simulink library "hdlcoderNFPCast"  (R2019a)
settings: Solver=VariableStepAuto  StartTime=0.0  StopTime=10.0  RelTol=1e-3
libraries: hdlsllib x7
settings Model: Creator=The MathWorks, Inc.  LastModifiedBy=The MathWorks, Inc.
settings DataIOCC: ReturnWorkspaceOutputs=off
settings DebuggingCC: ArithmeticOperatorsInVariantConditions=warning
settings SFSimCC: SimUseLocalCustomCode=off
settings RTWCC: RTWUseLocalCustomCode=off
settings CodeAppCC: StateflowObjectComments=on
settings GRTTargetCC: TargetLangStandard=C89/C90 (ANSI)
settings ConfigComp: CovMetricSettings=dsw  CovHtmlReporting=on  CovSaveCumulativeToWorkspaceVar=on  CovSaveSingleToWorkspaceVar=on  CovShowResultsExplorer=off  CovExternalEMLEnable=off

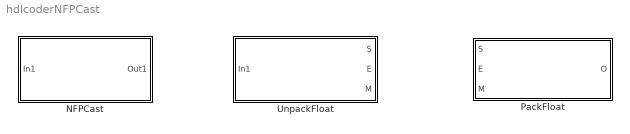
== system hdlcoderNFPCast ==
  NFPCast : Subsystem  mask(NFP Cast Operator){}
      mask help:
      | NFP Cast Operator casts from float to fixed and vice-versa.
      | - Integer input data type: uint32 and uint64 are supported.
      | - Floating-point input data type: single and double are supported.
      mask Display:
      | %image('blank_block.bmp')
      | color('darkBlue')
      | fprintf('Cast\n(Float <=> Fixed)')
      | port_label('input', 1, 'In')
      | port_label('output', 1, 'Out')
  PackFloat : Subsystem  mask(Pack Float){dataType=single}
      mask help:
      | Unpack Float to Sign, Exponent and Mantissa
      | - Input Data Type: fixed-point (S, E, M)
      | - Pop-up Mask: single or double
      | - Output Data Type: single or double
      mask init:
      | switch dataType
      |     case 'single'
      |         numbits = 32;
      |         manbits = 23;
      |     case 'double'
      |         numbits = 64;
      |         manbits = 52;
      |     otherwise
      |         assert(true);
      | end
      mask TypeOptions dataType: single | double
      mask Display:
      | %image('blank_block.bmp')
      | color('darkBlue')
      | fprintf('Pack\n<Float>')
      | port_label('input', 1, 'S')
      | port_label('input', 2, 'E')
      | port_label('input', 3, 'M')
      | port_label('output', 1, 'O')
  UnpackFloat : Subsystem  mask(Unpack Float){dataType=single}
      mask help:
      | Unpack Float to Sign, Exponent and Mantissa
      | - Input Data Type: single or double
      | - Pop-up Mask: single or double
      | - Output Data Type: fixed-point (S, E, M)
      mask init:
      | switch dataType
      |     case 'single'
      |         numbits = 32;
      |         manbits = 23;
      |     case 'double'
      |         numbits = 64;
      |         manbits = 52;
      |     otherwise
      |         assert(true);
      | end
      mask TypeOptions dataType: single | double
      mask Display:
      | %image('blank_block.bmp')
      | color('darkBlue')
      | fprintf('Unpack\n<Float>')
      | port_label('output', 1, 'S')
      | port_label('output', 2, 'E')
      | port_label('output', 3, 'M')
      | port_label('input', 1, 'In')

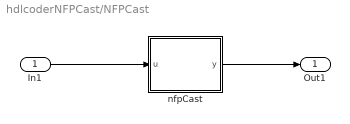
== system hdlcoderNFPCast/NFPCast ==
  In1 : Inport
  nfpCast : MATLAB Function  TreatAsAtomicUnit=on
  Out1 : Outport
  wires:
  nfpCast/1(y) -> Out1/1
  In1/1 -> nfpCast/1(u)

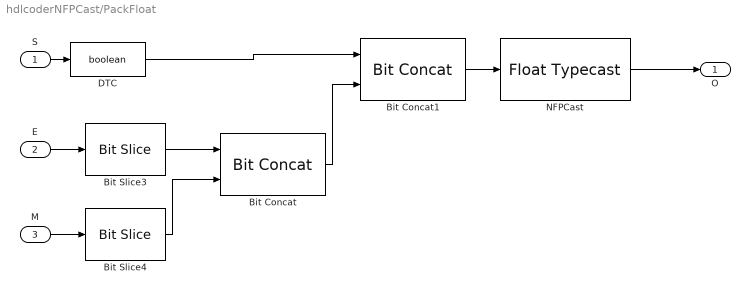
== system hdlcoderNFPCast/PackFloat ==
  S : Inport
  E : Inport  Port=2
  M : Inport  Port=3
  Bit Concat : hdlsllib/Logic and Bit Operations/Bit Concat  numInputs=2
      settings: SourceProductName=Simulink
  Bit Concat1 : hdlsllib/Logic and Bit Operations/Bit Concat  numInputs=2
      settings: SourceProductName=Simulink
  Bit Slice3 : hdlsllib/Logic and Bit Operations/Bit Slice  lidx=numbits-2 - manbits  ridx=0
      settings: SourceProductName=Simulink  SourceProductBaseCode=SL
  Bit Slice4 : hdlsllib/Logic and Bit Operations/Bit Slice  lidx=manbits-1  ridx=0
      settings: SourceProductName=Simulink  SourceProductBaseCode=SL
  DTC : DataTypeConversion  OutDataTypeStr=boolean
  NFPCast : FloatTypecast
  O : Outport
  wires:
  Bit Concat/1 -> Bit Concat1/2
  DTC/1 -> Bit Concat1/1
  Bit Concat1/1 -> NFPCast/1
  M/1 -> Bit Slice4/1
  E/1 -> Bit Slice3/1
  Bit Slice3/1 -> Bit Concat/1
  Bit Slice4/1 -> Bit Concat/2
  S/1 -> DTC/1
  NFPCast/1 -> O/1

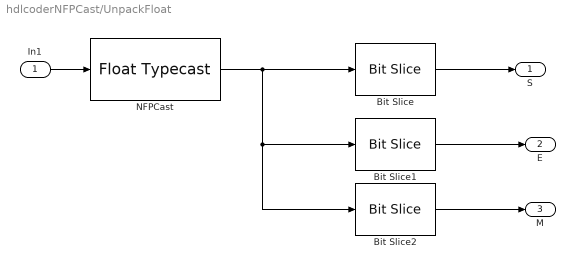
== system hdlcoderNFPCast/UnpackFloat ==
  In1 : Inport
  Bit Slice : hdlsllib/Logic and Bit Operations/Bit Slice  lidx=numbits-1  ridx=numbits-1
      settings: SourceProductName=Simulink  SourceProductBaseCode=SL
  Bit Slice1 : hdlsllib/Logic and Bit Operations/Bit Slice  lidx=numbits-2  ridx=manbits
      settings: SourceProductName=Simulink  SourceProductBaseCode=SL
  Bit Slice2 : hdlsllib/Logic and Bit Operations/Bit Slice  lidx=manbits-1  ridx=0
      settings: SourceProductName=Simulink  SourceProductBaseCode=SL
  NFPCast : FloatTypecast
  S : Outport
  E : Outport  Port=2
  M : Outport  Port=3
  wires:
  Bit Slice2/1 -> M/1
  In1/1 -> NFPCast/1
  Bit Slice1/1 -> E/1
  Bit Slice/1 -> S/1
  NFPCast/1 -> Bit Slice1/1, Bit Slice2/1, Bit Slice/1

== matlab function hdlcoderNFPCast/NFPCast/nfpCast ==
  data: u input; y output
function y = nfpCast(u)
coder.extrinsic('sprintf');
if isa(u, 'single')
    y = typecast(single(u), 'uint32');
elseif isa(u, 'double')
    fxp = fi(0, 0, 64, 0);
    interm = typecast(double(u), 'uint64');
    y = cast(interm, 'like', fxp);
elseif isa(u, 'uint32')
    y = typecast(u, 'single');
elseif isa(u, 'uint64')
    y = typecast(u, 'double');
elseif isa(u, 'embedded.fi')
    if (u.WordLength == 64) && strcmp(u.Signedness, 'Unsigned') && (u.FractionLength == 0)
        interm = uint64(u);
        y = typecast(interm, 'double');
    elseif (u.WordLength == 32) && strcmp(u.Signedness, 'Unsigned') && (u.FractionLength == 0)
        interm = uint32(u);
        y = typecast(interm, 'single');
    else
        y = cast(0, 'like', u);
        dtstr = sprintf('fixdt(%d,%d,%d)', ~strcmp(u.Signedness, 'Unsigned'), ...
                  u.WordLength, u.FractionLength);
        assert(false, ['Input data type: "' dtstr '" cannot be casted to float.']);
    end
else
    y = cast(0, 'like', u);
    assert(false, ['Input data type: "' class(u) '" cannot be casted to float.']);
end
end
